simulink model "GLIDESLOPEDIAGRAM"  (R2024a)
settings: Solver=VariableStepAuto  StartTime=0.0  StopTime=10.0  RelTol=1e-3
undefined symbols (not defined in the file or in its folder): magnitude
libraries: simulink_extras x1
settings Model: Creator=Aksha  LastModifiedBy=Aksha

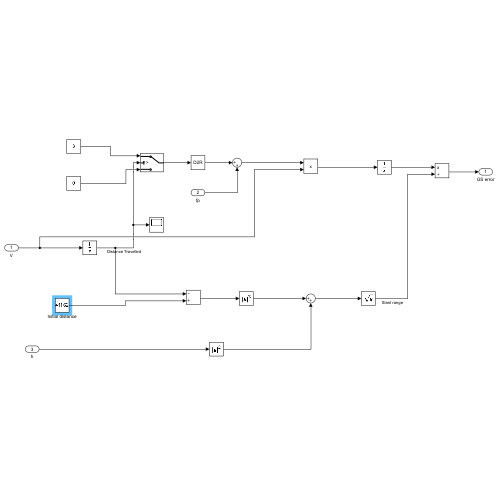
[thumbnail: Simulink's stored preview of the top-level diagram]
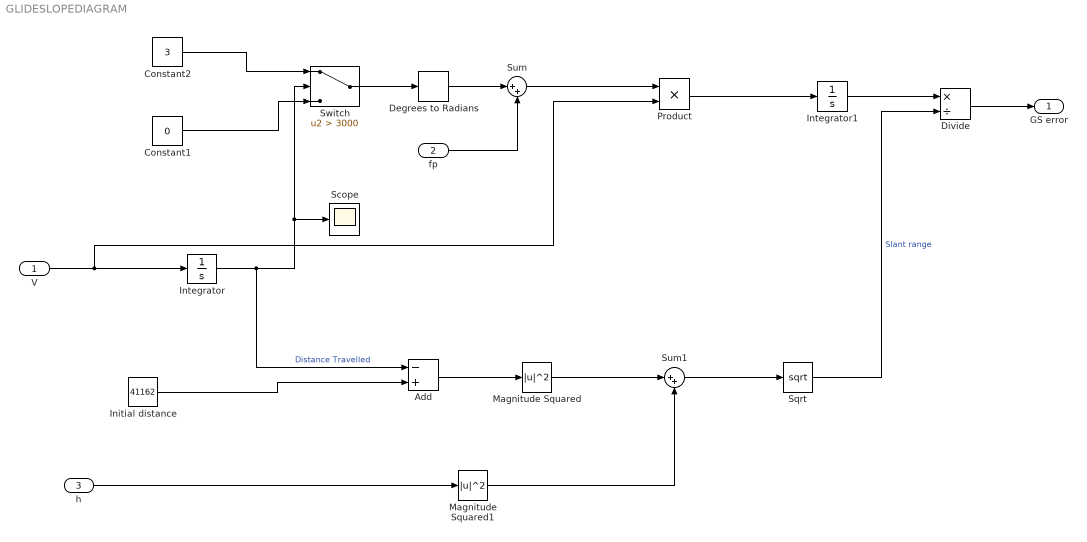
== system GLIDESLOPEDIAGRAM ==
  V : Inport
  fp : Inport  Port=2
  h : Inport  Port=3
  Add : Sum  Inputs=-+
  Constant1 : Constant  Value=0
  Constant2 : Constant  Value=3
  Degrees to Radians : simulink_extras/Transformations/Degrees to Radians
  Divide : Product  Inputs=*/
  Initial distance : Constant  Value=41162
  Integrator : Integrator
  Integrator1 : Integrator
  Magnitude Squared : Math  Operator=magnitude^2
  Magnitude Squared1 : Math  Operator=magnitude^2
  Product : Product
  Scope : Scope
  Sqrt : Sqrt
  Sum : Sum  Inputs=|++
  Sum1 : Sum  Inputs=|++
  Switch : Switch  Criteria=u2 > Threshold  Threshold=3000  SaturateOnIntegerOverflow=off  InputSameDT=off
  GS error : Outport
  wires:
  Constant2/1 -> Switch/1
  Constant1/1 -> Switch/3
  Integrator/1 -> Add/1, Switch/2, Scope/1  "Distance Travelled"
  Switch/1 -> Degrees to Radians/1
  Degrees to Radians/1 -> Sum/1
  Sum/1 -> Product/1
  Product/1 -> Integrator1/1
  Integrator1/1 -> Divide/1
  Add/1 -> Magnitude Squared/1
  Initial distance/1 -> Add/2
  Magnitude Squared/1 -> Sum1/1
  h/1 -> Magnitude Squared1/1
  Magnitude Squared1/1 -> Sum1/2
  Sum1/1 -> Sqrt/1
  Sqrt/1 -> Divide/2  "Slant range"
  V/1 -> Product/2, Integrator/1
  fp/1 -> Sum/2
  Divide/1 -> GS error/1
